simulink model "sin_with_name"  (R2023b)
settings: Solver=VariableStepAuto  StartTime=0.0  StopTime=32  RelTol=1e-3
libraries: simulink x1
settings Model: Creator=1234  LastModifiedBy=1234

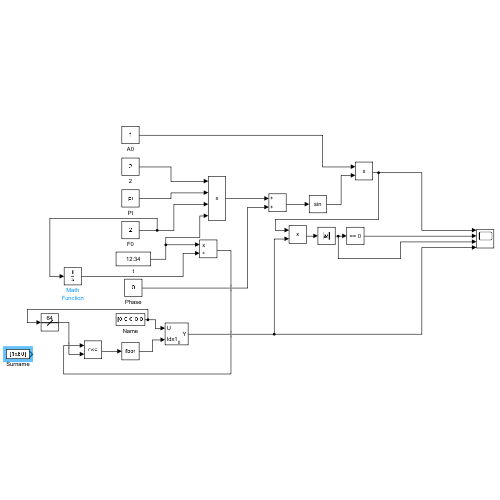
[thumbnail: Simulink's stored preview of the top-level diagram]
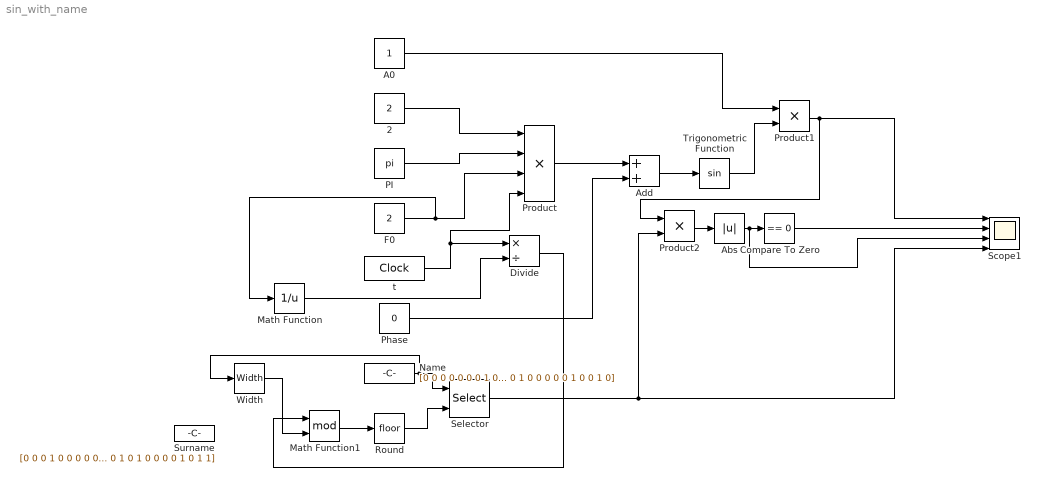
== system sin_with_name ==
  2 : Constant  Value=2
  A0 : Constant
  Abs : Abs  SaturateOnIntegerOverflow=off
  Add : Sum
  Compare To Zero : simulink/Logic and Bit Operations/Compare To Zero  relop===  OutDataTypeStr=boolean
  Divide : Product  Inputs=*/
  F0 : Constant  Value=2
  Math Function : Math  Operator=reciprocal
  Math Function1 : Math  Operator=mod
  Name : Constant  Value=[0 0 0 0 0 0 0 1 0 0 0 0 1 1 0 0 0 0 0 0 0 1 0 1 0 0 0 1 1 0 0 0 0 0 0 0 0 0 0 1 0 0 0 0 1 1 1 0 0 0 0 0 0 1 0 0 0 0 0 1 0 0 1 0]
  PI : Constant  Value=pi
  Phase : Constant  Value=0
  Product : Product  Inputs=4
  Product1 : Product
  Product2 : Product
  Round : Rounding
  Scope1 : Scope  NumInputPorts=4
  Selector : Selector  IndexMode=Zero-based  InputPortWidth=64  IndexOptions=Index vector (port)  Indices=[1 3]  OutputSizes=1
  Surname : Constant  Value=[0 0 0 1 0 0 0 0 0 0 0 0 1 1 1 1 0 0 0 0 0 1 1 1 0 0 0 1 0 0 1 0 0 0 0 0 0 1 0 1 0 0 0 0 0 0 1 0 0 0 0 0 1 1 1 0 0 0 0 1 1 0 0 1 0 0 0 1 0 1 0 1 0 0 0 0 1 0 1 1]
  Trigonometric Function : Trigonometry
  Width : Width
  t : DigitalClock  SampleTime=1/1000
  wires:
  2/1 -> Product/1
  PI/1 -> Product/2
  t/1 -> Product/4, Divide/1
  Phase/1 -> Add/2
  Add/1 -> Trigonometric Function/1
  Trigonometric Function/1 -> Product1/2
  A0/1 -> Product1/1
  Product1/1 -> Scope1/1, Product2/1
  Selector/1 -> Scope1/4, Product2/2
  Product/1 -> Add/1
  Math Function1/1 -> Round/1
  Round/1 -> Selector/2
  Product2/1 -> Abs/1
  Divide/1 -> Math Function1/1
  Abs/1 -> Scope1/3, Compare To Zero/1
  Compare To Zero/1 -> Scope1/2
  Name/1 -> Width/1, Selector/1
  Width/1 -> Math Function1/2
  Math Function/1 -> Divide/2
  F0/1 -> Math Function/1, Product/3
